simulink model "three_robot_cluster_all_primitives"  (R2024b)
settings: Solver=FixedStepDiscrete  StartTime=0.0  StopTime=60  FixedStep=0.1  MaxStep=0.1  RelTol=1e-3
libraries: neural x165, realtime_pacer_lib x1, simulink x1
(part 2 of 8)

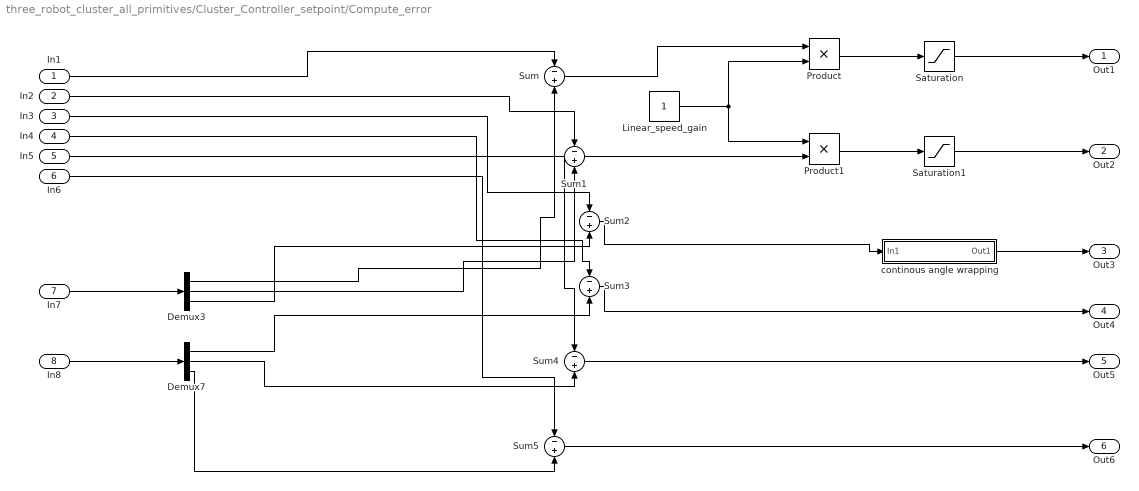
== system three_robot_cluster_all_primitives/Cluster_Controller_setpoint/Compute_error ==
  In1 : Inport
  In2 : Inport  Port=2
  In3 : Inport  Port=3
  In4 : Inport  Port=4
  In5 : Inport  Port=5
  In6 : Inport  Port=6
  In7 : Inport  Port=7
  In8 : Inport  Port=8
  Demux3 : Demux  Outputs=3
  Demux7 : Demux  Outputs=3
  Linear_speed_gain : Constant
  Product : Product
  Product1 : Product
  Saturation : Saturate  UpperLimit=0.3  LowerLimit=-0.3
  Saturation1 : Saturate  UpperLimit=0.3  LowerLimit=-0.3
  Sum{,1..5} (6 alike) : Sum  Inputs=-+
  continous angle wrapping : Subsystem
  Out1 : Outport
  Out2 : Outport  Port=2
  Out3 : Outport  Port=3
  Out4 : Outport  Port=4
  Out5 : Outport  Port=5
  Out6 : Outport  Port=6
  wires:
  In3/1 -> Sum2/1
  Demux3/2 -> Sum1/2
  Sum3/1 -> Out4/1
  In2/1 -> Sum1/1
  Demux3/3 -> Sum2/2
  Demux7/3 -> Sum5/2
  In8/1 -> Demux7/1
  Demux7/1 -> Sum3/2
  In1/1 -> Sum/1
  In5/1 -> Sum4/1
  Demux7/2 -> Sum4/2
  In6/1 -> Sum5/1
  Sum4/1 -> Out5/1
  Sum5/1 -> Out6/1
  Demux3/1 -> Sum/2
  In4/1 -> Sum3/1
  In7/1 -> Demux3/1
  Sum2/1 -> continous angle wrapping/1(In1)
  continous angle wrapping/1(Out1) -> Out3/1
  Sum/1 -> Product/1
  Linear_speed_gain/1 -> Product/2, Product1/1
  Sum1/1 -> Product1/2
  Saturation/1 -> Out1/1
  Product/1 -> Saturation/1
  Product1/1 -> Saturation1/1
  Saturation1/1 -> Out2/1

== system three_robot_cluster_all_primitives/Jacobian_primitive/Critical_point_predicter ==
  hue : Inport
  Sat : Inport  Port=2
  robot1 : Inport  Port=3
  robot2 : Inport  Port=4
  robot3 : Inport  Port=5
  Constant2 : Constant  Value=0
  Demux{,1..4} (5 alike) : Demux  Outputs=3
  Desired_set_point_Jacobian : ToWorkspace  VariableName=detected_critical_point  SampleTime=-1
  MATLAB Function : MATLAB Function  TreatAsAtomicUnit=on
  Sat_rescaling : Subsystem
  Subsystem : Subsystem
  Subsystem1 : Subsystem
  Subsystem2 : Subsystem
  Vector Concatenate : Concatenate
  x_desired : Outport
  y_desired : Outport  Port=2
  th_c_desired : Outport  Port=3
  wires:
  Vector Concatenate/1 -> Desired_set_point_Jacobian/1
  Constant2/1 -> th_c_desired/1
  Sat/1 -> Demux1/1
  hue/1 -> Demux/1
  Demux/1 -> Subsystem/1(hue)
  Demux/2 -> Subsystem1/1(hue)
  Demux/3 -> Subsystem2/1(hue)
  Demux1/1 -> Sat_rescaling/1(In1)
  Demux1/2 -> Sat_rescaling/2(In2)
  Demux1/3 -> Sat_rescaling/3(In3)
  Sat_rescaling/1(saturation) -> Subsystem/2(saturation)
  Sat_rescaling/2(saturation1) -> Subsystem1/2(saturation)
  Sat_rescaling/3(saturation2) -> Subsystem2/2(saturation)
  robot3/1 -> Demux4/1
  robot2/1 -> Demux3/1
  robot1/1 -> Demux2/1
  Subsystem/1(X_Component) -> MATLAB Function/3(u1)  "x_component"
  Subsystem/2(Y_Component) -> MATLAB Function/4(v1)  "y_component"
  Subsystem1/1(X_Component) -> MATLAB Function/7(u2)  "x_component"
  Subsystem1/2(Y_Component) -> MATLAB Function/8(v2)  "y_component"
  Subsystem2/1(X_Component) -> MATLAB Function/11(u3)  "x_component"
  Subsystem2/2(Y_Component) -> MATLAB Function/12(v3)  "y_component"
  Demux2/1 -> MATLAB Function/1(x1)
  Demux2/2 -> MATLAB Function/2(y1)
  Demux3/1 -> MATLAB Function/5(x2)
  Demux3/2 -> MATLAB Function/6(y2)
  Demux4/1 -> MATLAB Function/9(x3)
  Demux4/2 -> MATLAB Function/10(y3)
  MATLAB Function/1(x) -> Vector Concatenate/1, x_desired/1
  MATLAB Function/2(y) -> y_desired/1, Vector Concatenate/2

== system three_robot_cluster_all_primitives/Jacobian_primitive/formation_error ==
  a : Inport
  b : Inport  Port=2
  c : Inport  Port=3
  a,b,c desired : Inport  Port=4
  Demux7 : Demux  Outputs=3
  Sum3 : Sum  Inputs=-+
  Sum4 : Sum  Inputs=-+
  Sum5 : Sum  Inputs=-+
  a_err : Outport
  b_err : Outport  Port=2
  C_err : Outport  Port=3
  wires:
  Sum3/1 -> a_err/1
  Demux7/3 -> Sum5/2
  a,b,c desired/1 -> Demux7/1
  Demux7/1 -> Sum3/2
  b/1 -> Sum4/1
  Demux7/2 -> Sum4/2
  c/1 -> Sum5/1
  Sum4/1 -> b_err/1
  Sum5/1 -> C_err/1
  a/1 -> Sum3/1

== system three_robot_cluster_all_primitives/Jacobian_primitive/position_error ==
  x_c : Inport
  y_c : Inport  Port=2
  th_c : Inport  Port=3
  x,y,thC desired : Inport  Port=4
  Constant : Constant
  Demux7 : Demux  Outputs=3
  Product : Product
  Product1 : Product
  Saturation : Saturate  UpperLimit=0.3  LowerLimit=-0.3
  Saturation1 : Saturate  UpperLimit=0.3  LowerLimit=-0.3
  Sum3 : Sum  Inputs=-+
  Sum4 : Sum  Inputs=-+
  Sum5 : Sum  Inputs=-+
  thC_err : Outport
  xc_err : Outport  Port=2
  yc_err : Outport  Port=3
  wires:
  Demux7/3 -> Sum5/2
  x,y,thC desired/1 -> Demux7/1
  Demux7/1 -> Sum3/2
  y_c/1 -> Sum4/1
  Demux7/2 -> Sum4/2
  th_c/1 -> Sum5/1
  Sum5/1 -> thC_err/1
  x_c/1 -> Sum3/1
  Constant/1 -> Product1/1, Product/1
  Sum3/1 -> Product/2
  Sum4/1 -> Product1/2
  Saturation/1 -> xc_err/1
  Product/1 -> Saturation/1
  Saturation1/1 -> yc_err/1
  Product1/1 -> Saturation1/1

== system three_robot_cluster_all_primitives/RGB to HSV to vel - all robots/Hue Neural Network ==
  Input : Inport  PortDimensions=4
      mask Display: e = 0.06;c1 = [120 230 180]/255;c2 = ([120 230 180]+0)/(256+128);c3 = ([120 230 180]+128)/(256+128);patch([0 1 1 0],[0 0 1 1],c1);patch([0 1 1 1-e 1-e 0+e],[0 0 1 1-e 0+e 0+e],c2);patch([0 0 1 1-e 0+e 0+e],[0 1 1 1-e 1-e 0+e],c3);plot([0 1 1 0 0],[0 0 1 1 0]);
  Layer 1 : Subsystem
      mask Display: e = 0.06;c1 = [120 150 230]/255;c2 = ([120 150 230]+0)/383;c3 = ([120 150 230]+128)/383;patch([0 1 1 0],[0 0 1 1],c1);patch([0 1 1 1-e 1-e 0+e],[0 0 1 1-e 0+e 0+e],c2);patch([0 0 1 1-e 0+e 0+e],[0 1 1 1-e 1-e 0+e],c3);plot([0 1 1 0 0],[0 0 1 1 0]);
  Layer 2 : Subsystem
      mask Display: e = 0.06;c1 = [120 150 230]/255;c2 = ([120 150 230]+0)/383;c3 = ([120 150 230]+128)/383;patch([0 1 1 0],[0 0 1 1],c1);patch([0 1 1 1-e 1-e 0+e],[0 0 1 1-e 0+e 0+e],c2);patch([0 0 1 1-e 0+e 0+e],[0 1 1 1-e 1-e 0+e],c3);plot([0 1 1 0 0],[0 0 1 1 0]);
  Layer 3 : Subsystem
      mask Display: e = 0.06;c1 = [120 150 230]/255;c2 = ([120 150 230]+0)/383;c3 = ([120 150 230]+128)/383;patch([0 1 1 0],[0 0 1 1],c1);patch([0 1 1 1-e 1-e 0+e],[0 0 1 1-e 0+e 0+e],c2);patch([0 0 1 1-e 0+e 0+e],[0 1 1 1-e 1-e 0+e],c3);plot([0 1 1 0 0],[0 0 1 1 0]);
  Process Input 1 : Subsystem
      mask Display: e = 0.06;c1 = [120 150 230]/255;c2 = ([120 150 230]+0)/383;c3 = ([120 150 230]+128)/383;patch([0 1 1 0],[0 0 1 1],c1);patch([0 1 1 1-e 1-e 0+e],[0 0 1 1-e 0+e 0+e],c2);patch([0 0 1 1-e 0+e 0+e],[0 1 1 1-e 1-e 0+e],c3);plot([0 1 1 0 0],[0 0 1 1 0]);
  Process Output 1 : Subsystem
      mask Display: e = 0.06;c1 = [120 150 230]/255;c2 = ([120 150 230]+0)/383;c3 = ([120 150 230]+128)/383;patch([0 1 1 0],[0 0 1 1],c1);patch([0 1 1 1-e 1-e 0+e],[0 0 1 1-e 0+e 0+e],c2);patch([0 0 1 1-e 0+e 0+e],[0 1 1 1-e 1-e 0+e],c3);plot([0 1 1 0 0],[0 0 1 1 0]);
  Output : Outport  InitialOutput=[0;0]
      mask Display: e = 0.06;c1 = [120 230 180]/255;c2 = ([120 230 180]+0)/(256+128);c3 = ([120 230 180]+128)/(256+128);patch([0 1 1 0],[0 0 1 1],c1);patch([0 1 1 1-e 1-e 0+e],[0 0 1 1-e 0+e 0+e],c2);patch([0 0 1 1-e 0+e 0+e],[0 1 1 1-e 1-e 0+e],c3);plot([0 1 1 0 0],[0 0 1 1 0]);
  wires:
  Input/1 -> Process Input 1/1(x)
  Process Output 1/1(y) -> Output/1
  Process Input 1/1(p) -> Layer 1/1("p{1}")
  Layer 1/1("a{1}") -> [feedback1]
  [feedback1] -> Layer 2/1("a{1} ")
  Layer 2/1("a{2}") -> [feedback2]
  [feedback2] -> Layer 3/1("a{2} ")
  Layer 3/1("a{3}") -> Process Output 1/1(a)

== system three_robot_cluster_all_primitives/RGB to HSV to vel - all robots/Sat Neural Network ==
  Input : Inport  PortDimensions=4
      mask Display: e = 0.06;c1 = [120 230 180]/255;c2 = ([120 230 180]+0)/(256+128);c3 = ([120 230 180]+128)/(256+128);patch([0 1 1 0],[0 0 1 1],c1);patch([0 1 1 1-e 1-e 0+e],[0 0 1 1-e 0+e 0+e],c2);patch([0 0 1 1-e 0+e 0+e],[0 1 1 1-e 1-e 0+e],c3);plot([0 1 1 0 0],[0 0 1 1 0]);
  Layer 1 : Subsystem
      mask Display: e = 0.06;c1 = [120 150 230]/255;c2 = ([120 150 230]+0)/383;c3 = ([120 150 230]+128)/383;patch([0 1 1 0],[0 0 1 1],c1);patch([0 1 1 1-e 1-e 0+e],[0 0 1 1-e 0+e 0+e],c2);patch([0 0 1 1-e 0+e 0+e],[0 1 1 1-e 1-e 0+e],c3);plot([0 1 1 0 0],[0 0 1 1 0]);
  Layer 2 : Subsystem
      mask Display: e = 0.06;c1 = [120 150 230]/255;c2 = ([120 150 230]+0)/383;c3 = ([120 150 230]+128)/383;patch([0 1 1 0],[0 0 1 1],c1);patch([0 1 1 1-e 1-e 0+e],[0 0 1 1-e 0+e 0+e],c2);patch([0 0 1 1-e 0+e 0+e],[0 1 1 1-e 1-e 0+e],c3);plot([0 1 1 0 0],[0 0 1 1 0]);
  Layer 3 : Subsystem
      mask Display: e = 0.06;c1 = [120 150 230]/255;c2 = ([120 150 230]+0)/383;c3 = ([120 150 230]+128)/383;patch([0 1 1 0],[0 0 1 1],c1);patch([0 1 1 1-e 1-e 0+e],[0 0 1 1-e 0+e 0+e],c2);patch([0 0 1 1-e 0+e 0+e],[0 1 1 1-e 1-e 0+e],c3);plot([0 1 1 0 0],[0 0 1 1 0]);
  Process Input 1 : Subsystem
      mask Display: e = 0.06;c1 = [120 150 230]/255;c2 = ([120 150 230]+0)/383;c3 = ([120 150 230]+128)/383;patch([0 1 1 0],[0 0 1 1],c1);patch([0 1 1 1-e 1-e 0+e],[0 0 1 1-e 0+e 0+e],c2);patch([0 0 1 1-e 0+e 0+e],[0 1 1 1-e 1-e 0+e],c3);plot([0 1 1 0 0],[0 0 1 1 0]);
  Process Output 1 : Subsystem
      mask Display: e = 0.06;c1 = [120 150 230]/255;c2 = ([120 150 230]+0)/383;c3 = ([120 150 230]+128)/383;patch([0 1 1 0],[0 0 1 1],c1);patch([0 1 1 1-e 1-e 0+e],[0 0 1 1-e 0+e 0+e],c2);patch([0 0 1 1-e 0+e 0+e],[0 1 1 1-e 1-e 0+e],c3);plot([0 1 1 0 0],[0 0 1 1 0]);
  Output : Outport  InitialOutput=0
      mask Display: e = 0.06;c1 = [120 230 180]/255;c2 = ([120 230 180]+0)/(256+128);c3 = ([120 230 180]+128)/(256+128);patch([0 1 1 0],[0 0 1 1],c1);patch([0 1 1 1-e 1-e 0+e],[0 0 1 1-e 0+e 0+e],c2);patch([0 0 1 1-e 0+e 0+e],[0 1 1 1-e 1-e 0+e],c3);plot([0 1 1 0 0],[0 0 1 1 0]);
  wires:
  Input/1 -> Process Input 1/1(x)
  Process Output 1/1(y) -> Output/1
  Process Input 1/1(p) -> Layer 1/1("p{1}")
  Layer 1/1("a{1}") -> [feedback1]
  [feedback1] -> Layer 2/1("a{1} ")
  Layer 2/1("a{2}") -> [feedback2]
  [feedback2] -> Layer 3/1("a{2} ")
  Layer 3/1("a{3}") -> Process Output 1/1(a)

== system three_robot_cluster_all_primitives/RGB to HSV to vel - all robots1/Hue Neural Network ==
  Input : Inport  PortDimensions=4
      mask Display: e = 0.06;c1 = [120 230 180]/255;c2 = ([120 230 180]+0)/(256+128);c3 = ([120 230 180]+128)/(256+128);patch([0 1 1 0],[0 0 1 1],c1);patch([0 1 1 1-e 1-e 0+e],[0 0 1 1-e 0+e 0+e],c2);patch([0 0 1 1-e 0+e 0+e],[0 1 1 1-e 1-e 0+e],c3);plot([0 1 1 0 0],[0 0 1 1 0]);
  Layer 1 : Subsystem
      mask Display: e = 0.06;c1 = [120 150 230]/255;c2 = ([120 150 230]+0)/383;c3 = ([120 150 230]+128)/383;patch([0 1 1 0],[0 0 1 1],c1);patch([0 1 1 1-e 1-e 0+e],[0 0 1 1-e 0+e 0+e],c2);patch([0 0 1 1-e 0+e 0+e],[0 1 1 1-e 1-e 0+e],c3);plot([0 1 1 0 0],[0 0 1 1 0]);
  Layer 2 : Subsystem
      mask Display: e = 0.06;c1 = [120 150 230]/255;c2 = ([120 150 230]+0)/383;c3 = ([120 150 230]+128)/383;patch([0 1 1 0],[0 0 1 1],c1);patch([0 1 1 1-e 1-e 0+e],[0 0 1 1-e 0+e 0+e],c2);patch([0 0 1 1-e 0+e 0+e],[0 1 1 1-e 1-e 0+e],c3);plot([0 1 1 0 0],[0 0 1 1 0]);
  Layer 3 : Subsystem
      mask Display: e = 0.06;c1 = [120 150 230]/255;c2 = ([120 150 230]+0)/383;c3 = ([120 150 230]+128)/383;patch([0 1 1 0],[0 0 1 1],c1);patch([0 1 1 1-e 1-e 0+e],[0 0 1 1-e 0+e 0+e],c2);patch([0 0 1 1-e 0+e 0+e],[0 1 1 1-e 1-e 0+e],c3);plot([0 1 1 0 0],[0 0 1 1 0]);
  Process Input 1 : Subsystem
      mask Display: e = 0.06;c1 = [120 150 230]/255;c2 = ([120 150 230]+0)/383;c3 = ([120 150 230]+128)/383;patch([0 1 1 0],[0 0 1 1],c1);patch([0 1 1 1-e 1-e 0+e],[0 0 1 1-e 0+e 0+e],c2);patch([0 0 1 1-e 0+e 0+e],[0 1 1 1-e 1-e 0+e],c3);plot([0 1 1 0 0],[0 0 1 1 0]);
  Process Output 1 : Subsystem
      mask Display: e = 0.06;c1 = [120 150 230]/255;c2 = ([120 150 230]+0)/383;c3 = ([120 150 230]+128)/383;patch([0 1 1 0],[0 0 1 1],c1);patch([0 1 1 1-e 1-e 0+e],[0 0 1 1-e 0+e 0+e],c2);patch([0 0 1 1-e 0+e 0+e],[0 1 1 1-e 1-e 0+e],c3);plot([0 1 1 0 0],[0 0 1 1 0]);
  Output : Outport  InitialOutput=[0;0]
      mask Display: e = 0.06;c1 = [120 230 180]/255;c2 = ([120 230 180]+0)/(256+128);c3 = ([120 230 180]+128)/(256+128);patch([0 1 1 0],[0 0 1 1],c1);patch([0 1 1 1-e 1-e 0+e],[0 0 1 1-e 0+e 0+e],c2);patch([0 0 1 1-e 0+e 0+e],[0 1 1 1-e 1-e 0+e],c3);plot([0 1 1 0 0],[0 0 1 1 0]);
  wires:
  Input/1 -> Process Input 1/1(x)
  Process Output 1/1(y) -> Output/1
  Process Input 1/1(p) -> Layer 1/1("p{1}")
  Layer 1/1("a{1}") -> [feedback1]
  [feedback1] -> Layer 2/1("a{1} ")
  Layer 2/1("a{2}") -> [feedback2]
  [feedback2] -> Layer 3/1("a{2} ")
  Layer 3/1("a{3}") -> Process Output 1/1(a)

== system three_robot_cluster_all_primitives/RGB to HSV to vel - all robots1/Sat Neural Network ==
  Input : Inport  PortDimensions=4
      mask Display: e = 0.06;c1 = [120 230 180]/255;c2 = ([120 230 180]+0)/(256+128);c3 = ([120 230 180]+128)/(256+128);patch([0 1 1 0],[0 0 1 1],c1);patch([0 1 1 1-e 1-e 0+e],[0 0 1 1-e 0+e 0+e],c2);patch([0 0 1 1-e 0+e 0+e],[0 1 1 1-e 1-e 0+e],c3);plot([0 1 1 0 0],[0 0 1 1 0]);
  Layer 1 : Subsystem
      mask Display: e = 0.06;c1 = [120 150 230]/255;c2 = ([120 150 230]+0)/383;c3 = ([120 150 230]+128)/383;patch([0 1 1 0],[0 0 1 1],c1);patch([0 1 1 1-e 1-e 0+e],[0 0 1 1-e 0+e 0+e],c2);patch([0 0 1 1-e 0+e 0+e],[0 1 1 1-e 1-e 0+e],c3);plot([0 1 1 0 0],[0 0 1 1 0]);
  Layer 2 : Subsystem
      mask Display: e = 0.06;c1 = [120 150 230]/255;c2 = ([120 150 230]+0)/383;c3 = ([120 150 230]+128)/383;patch([0 1 1 0],[0 0 1 1],c1);patch([0 1 1 1-e 1-e 0+e],[0 0 1 1-e 0+e 0+e],c2);patch([0 0 1 1-e 0+e 0+e],[0 1 1 1-e 1-e 0+e],c3);plot([0 1 1 0 0],[0 0 1 1 0]);
  Layer 3 : Subsystem
      mask Display: e = 0.06;c1 = [120 150 230]/255;c2 = ([120 150 230]+0)/383;c3 = ([120 150 230]+128)/383;patch([0 1 1 0],[0 0 1 1],c1);patch([0 1 1 1-e 1-e 0+e],[0 0 1 1-e 0+e 0+e],c2);patch([0 0 1 1-e 0+e 0+e],[0 1 1 1-e 1-e 0+e],c3);plot([0 1 1 0 0],[0 0 1 1 0]);
  Process Input 1 : Subsystem
      mask Display: e = 0.06;c1 = [120 150 230]/255;c2 = ([120 150 230]+0)/383;c3 = ([120 150 230]+128)/383;patch([0 1 1 0],[0 0 1 1],c1);patch([0 1 1 1-e 1-e 0+e],[0 0 1 1-e 0+e 0+e],c2);patch([0 0 1 1-e 0+e 0+e],[0 1 1 1-e 1-e 0+e],c3);plot([0 1 1 0 0],[0 0 1 1 0]);
  Process Output 1 : Subsystem
      mask Display: e = 0.06;c1 = [120 150 230]/255;c2 = ([120 150 230]+0)/383;c3 = ([120 150 230]+128)/383;patch([0 1 1 0],[0 0 1 1],c1);patch([0 1 1 1-e 1-e 0+e],[0 0 1 1-e 0+e 0+e],c2);patch([0 0 1 1-e 0+e 0+e],[0 1 1 1-e 1-e 0+e],c3);plot([0 1 1 0 0],[0 0 1 1 0]);
  Output : Outport  InitialOutput=0
      mask Display: e = 0.06;c1 = [120 230 180]/255;c2 = ([120 230 180]+0)/(256+128);c3 = ([120 230 180]+128)/(256+128);patch([0 1 1 0],[0 0 1 1],c1);patch([0 1 1 1-e 1-e 0+e],[0 0 1 1-e 0+e 0+e],c2);patch([0 0 1 1-e 0+e 0+e],[0 1 1 1-e 1-e 0+e],c3);plot([0 1 1 0 0],[0 0 1 1 0]);
  wires:
  Input/1 -> Process Input 1/1(x)
  Process Output 1/1(y) -> Output/1
  Process Input 1/1(p) -> Layer 1/1("p{1}")
  Layer 1/1("a{1}") -> [feedback1]
  [feedback1] -> Layer 2/1("a{1} ")
  Layer 2/1("a{2}") -> [feedback2]
  [feedback2] -> Layer 3/1("a{2} ")
  Layer 3/1("a{3}") -> Process Output 1/1(a)

== system three_robot_cluster_all_primitives/RGB to HSV to vel - all robots2/Hue Neural Network ==
  Input : Inport  PortDimensions=4
      mask Display: e = 0.06;c1 = [120 230 180]/255;c2 = ([120 230 180]+0)/(256+128);c3 = ([120 230 180]+128)/(256+128);patch([0 1 1 0],[0 0 1 1],c1);patch([0 1 1 1-e 1-e 0+e],[0 0 1 1-e 0+e 0+e],c2);patch([0 0 1 1-e 0+e 0+e],[0 1 1 1-e 1-e 0+e],c3);plot([0 1 1 0 0],[0 0 1 1 0]);
  Layer 1 : Subsystem
      mask Display: e = 0.06;c1 = [120 150 230]/255;c2 = ([120 150 230]+0)/383;c3 = ([120 150 230]+128)/383;patch([0 1 1 0],[0 0 1 1],c1);patch([0 1 1 1-e 1-e 0+e],[0 0 1 1-e 0+e 0+e],c2);patch([0 0 1 1-e 0+e 0+e],[0 1 1 1-e 1-e 0+e],c3);plot([0 1 1 0 0],[0 0 1 1 0]);
  Layer 2 : Subsystem
      mask Display: e = 0.06;c1 = [120 150 230]/255;c2 = ([120 150 230]+0)/383;c3 = ([120 150 230]+128)/383;patch([0 1 1 0],[0 0 1 1],c1);patch([0 1 1 1-e 1-e 0+e],[0 0 1 1-e 0+e 0+e],c2);patch([0 0 1 1-e 0+e 0+e],[0 1 1 1-e 1-e 0+e],c3);plot([0 1 1 0 0],[0 0 1 1 0]);
  Layer 3 : Subsystem
      mask Display: e = 0.06;c1 = [120 150 230]/255;c2 = ([120 150 230]+0)/383;c3 = ([120 150 230]+128)/383;patch([0 1 1 0],[0 0 1 1],c1);patch([0 1 1 1-e 1-e 0+e],[0 0 1 1-e 0+e 0+e],c2);patch([0 0 1 1-e 0+e 0+e],[0 1 1 1-e 1-e 0+e],c3);plot([0 1 1 0 0],[0 0 1 1 0]);
  Process Input 1 : Subsystem
      mask Display: e = 0.06;c1 = [120 150 230]/255;c2 = ([120 150 230]+0)/383;c3 = ([120 150 230]+128)/383;patch([0 1 1 0],[0 0 1 1],c1);patch([0 1 1 1-e 1-e 0+e],[0 0 1 1-e 0+e 0+e],c2);patch([0 0 1 1-e 0+e 0+e],[0 1 1 1-e 1-e 0+e],c3);plot([0 1 1 0 0],[0 0 1 1 0]);
  Process Output 1 : Subsystem
      mask Display: e = 0.06;c1 = [120 150 230]/255;c2 = ([120 150 230]+0)/383;c3 = ([120 150 230]+128)/383;patch([0 1 1 0],[0 0 1 1],c1);patch([0 1 1 1-e 1-e 0+e],[0 0 1 1-e 0+e 0+e],c2);patch([0 0 1 1-e 0+e 0+e],[0 1 1 1-e 1-e 0+e],c3);plot([0 1 1 0 0],[0 0 1 1 0]);
  Output : Outport  InitialOutput=[0;0]
      mask Display: e = 0.06;c1 = [120 230 180]/255;c2 = ([120 230 180]+0)/(256+128);c3 = ([120 230 180]+128)/(256+128);patch([0 1 1 0],[0 0 1 1],c1);patch([0 1 1 1-e 1-e 0+e],[0 0 1 1-e 0+e 0+e],c2);patch([0 0 1 1-e 0+e 0+e],[0 1 1 1-e 1-e 0+e],c3);plot([0 1 1 0 0],[0 0 1 1 0]);
  wires:
  Input/1 -> Process Input 1/1(x)
  Process Output 1/1(y) -> Output/1
  Process Input 1/1(p) -> Layer 1/1("p{1}")
  Layer 1/1("a{1}") -> [feedback1]
  [feedback1] -> Layer 2/1("a{1} ")
  Layer 2/1("a{2}") -> [feedback2]
  [feedback2] -> Layer 3/1("a{2} ")
  Layer 3/1("a{3}") -> Process Output 1/1(a)

== system three_robot_cluster_all_primitives/RGB to HSV to vel - all robots2/Sat Neural Network ==
  Input : Inport  PortDimensions=4
      mask Display: e = 0.06;c1 = [120 230 180]/255;c2 = ([120 230 180]+0)/(256+128);c3 = ([120 230 180]+128)/(256+128);patch([0 1 1 0],[0 0 1 1],c1);patch([0 1 1 1-e 1-e 0+e],[0 0 1 1-e 0+e 0+e],c2);patch([0 0 1 1-e 0+e 0+e],[0 1 1 1-e 1-e 0+e],c3);plot([0 1 1 0 0],[0 0 1 1 0]);
  Layer 1 : Subsystem
      mask Display: e = 0.06;c1 = [120 150 230]/255;c2 = ([120 150 230]+0)/383;c3 = ([120 150 230]+128)/383;patch([0 1 1 0],[0 0 1 1],c1);patch([0 1 1 1-e 1-e 0+e],[0 0 1 1-e 0+e 0+e],c2);patch([0 0 1 1-e 0+e 0+e],[0 1 1 1-e 1-e 0+e],c3);plot([0 1 1 0 0],[0 0 1 1 0]);
  Layer 2 : Subsystem
      mask Display: e = 0.06;c1 = [120 150 230]/255;c2 = ([120 150 230]+0)/383;c3 = ([120 150 230]+128)/383;patch([0 1 1 0],[0 0 1 1],c1);patch([0 1 1 1-e 1-e 0+e],[0 0 1 1-e 0+e 0+e],c2);patch([0 0 1 1-e 0+e 0+e],[0 1 1 1-e 1-e 0+e],c3);plot([0 1 1 0 0],[0 0 1 1 0]);
  Layer 3 : Subsystem
      mask Display: e = 0.06;c1 = [120 150 230]/255;c2 = ([120 150 230]+0)/383;c3 = ([120 150 230]+128)/383;patch([0 1 1 0],[0 0 1 1],c1);patch([0 1 1 1-e 1-e 0+e],[0 0 1 1-e 0+e 0+e],c2);patch([0 0 1 1-e 0+e 0+e],[0 1 1 1-e 1-e 0+e],c3);plot([0 1 1 0 0],[0 0 1 1 0]);
  Process Input 1 : Subsystem
      mask Display: e = 0.06;c1 = [120 150 230]/255;c2 = ([120 150 230]+0)/383;c3 = ([120 150 230]+128)/383;patch([0 1 1 0],[0 0 1 1],c1);patch([0 1 1 1-e 1-e 0+e],[0 0 1 1-e 0+e 0+e],c2);patch([0 0 1 1-e 0+e 0+e],[0 1 1 1-e 1-e 0+e],c3);plot([0 1 1 0 0],[0 0 1 1 0]);
  Process Output 1 : Subsystem
      mask Display: e = 0.06;c1 = [120 150 230]/255;c2 = ([120 150 230]+0)/383;c3 = ([120 150 230]+128)/383;patch([0 1 1 0],[0 0 1 1],c1);patch([0 1 1 1-e 1-e 0+e],[0 0 1 1-e 0+e 0+e],c2);patch([0 0 1 1-e 0+e 0+e],[0 1 1 1-e 1-e 0+e],c3);plot([0 1 1 0 0],[0 0 1 1 0]);
  Output : Outport  InitialOutput=0
      mask Display: e = 0.06;c1 = [120 230 180]/255;c2 = ([120 230 180]+0)/(256+128);c3 = ([120 230 180]+128)/(256+128);patch([0 1 1 0],[0 0 1 1],c1);patch([0 1 1 1-e 1-e 0+e],[0 0 1 1-e 0+e 0+e],c2);patch([0 0 1 1-e 0+e 0+e],[0 1 1 1-e 1-e 0+e],c3);plot([0 1 1 0 0],[0 0 1 1 0]);
  wires:
  Input/1 -> Process Input 1/1(x)
  Process Output 1/1(y) -> Output/1
  Process Input 1/1(p) -> Layer 1/1("p{1}")
  Layer 1/1("a{1}") -> [feedback1]
  [feedback1] -> Layer 2/1("a{1} ")
  Layer 2/1("a{2}") -> [feedback2]
  [feedback2] -> Layer 3/1("a{2} ")
  Layer 3/1("a{3}") -> Process Output 1/1(a)

== system three_robot_cluster_all_primitives/vector2scalar_mag_steepest_ascent/3_robot HSV to vector ==
  Sat : Inport
  Robot_1_pose : Inport  Port=2
  robot_2_pose : Inport  Port=3
  robot_3_pose : Inport  Port=4
  Constant2 : Constant  Value=0
  Demux{,1..3} (4 alike) : Demux  Outputs=3
  Desired_velocities_new_primitve : ToWorkspace  VariableName=desired_velocities_gradient_descent  SampleTime=-1
  MATLAB Function : MATLAB Function  TreatAsAtomicUnit=on
  Scope : Scope  NumInputPorts=2
  Scope1 : Scope  NumInputPorts=2
  Scope2 : Scope  NumInputPorts=3
  Vector Concatenate : Concatenate  NumInputs=3
  y_velocity : Outport
  x_velocity : Outport  Port=2
  th_c velocity : Outport  Port=3
  wires:
  Vector Concatenate/1 -> Desired_velocities_new_primitve/1
  Constant2/1 -> th_c velocity/1, Vector Concatenate/3
  Sat/1 -> Demux/1
  Robot_1_pose/1 -> Demux1/1
  robot_2_pose/1 -> Demux2/1
  robot_3_pose/1 -> Demux3/1
  Demux1/1 -> Scope1/1, MATLAB Function/1(x1)
  Demux1/2 -> MATLAB Function/2(y1), Scope1/2
  Demux/1 -> Scope2/1, MATLAB Function/3(z1)
  Demux2/1 -> MATLAB Function/4(x2)
  Demux2/2 -> MATLAB Function/5(y2)
  Demux/2 -> Scope2/2, MATLAB Function/6(z2)
  Demux3/1 -> MATLAB Function/7(x3)
  Demux3/2 -> MATLAB Function/8(y3)
  Demux/3 -> Scope2/3, MATLAB Function/9(z3)
  MATLAB Function/1(x) -> Scope/1, x_velocity/1, Vector Concatenate/1
  MATLAB Function/2(y) -> Scope/2, y_velocity/1, Vector Concatenate/2

== system three_robot_cluster_all_primitives/vector2scalar_mag_steepest_ascent/formation_error ==
  a : Inport
  b : Inport  Port=2
  c : Inport  Port=3
  a,b,c desired : Inport  Port=4
  Demux7 : Demux  Outputs=3
  Sum3 : Sum  Inputs=-+
  Sum4 : Sum  Inputs=-+
  Sum5 : Sum  Inputs=-+
  Out4 : Outport
  Out5 : Outport  Port=2
  Out6 : Outport  Port=3
  wires:
  Sum3/1 -> Out4/1
  Demux7/3 -> Sum5/2
  a,b,c desired/1 -> Demux7/1
  Demux7/1 -> Sum3/2
  b/1 -> Sum4/1
  Demux7/2 -> Sum4/2
  c/1 -> Sum5/1
  Sum4/1 -> Out5/1
  Sum5/1 -> Out6/1
  a/1 -> Sum3/1

== system three_robot_cluster_all_primitives/vector2scalar_mag_steepest_descent/3_robot HSV to vector ==
  Sat : Inport
  Robot_1_pose : Inport  Port=2
  robot_2_pose : Inport  Port=3
  robot_3_pose : Inport  Port=4
  Constant2 : Constant  Value=0
  Demux{,1..3} (4 alike) : Demux  Outputs=3
  MATLAB Function : MATLAB Function  TreatAsAtomicUnit=on
  Scope : Scope  NumInputPorts=2
  Scope1 : Scope  NumInputPorts=2
  Scope2 : Scope  NumInputPorts=2
  x_velocity : Outport
  th_c velocity : Outport  Port=2
  y_velocity : Outport  Port=3
  wires:
  Constant2/1 -> th_c velocity/1
  Sat/1 -> Demux/1
  Robot_1_pose/1 -> Demux1/1
  robot_2_pose/1 -> Demux2/1
  robot_3_pose/1 -> Demux3/1
  Demux1/1 -> Scope1/1, MATLAB Function/1(x1)
  Demux1/2 -> MATLAB Function/2(y1), Scope1/2
  Demux/1 -> Scope2/1, MATLAB Function/3(z1)
  Demux2/1 -> MATLAB Function/4(x2)
  Demux2/2 -> MATLAB Function/5(y2)
  Demux/2 -> Scope2/2, MATLAB Function/6(z2)
  Demux3/1 -> MATLAB Function/7(x3)
  Demux3/2 -> MATLAB Function/8(y3)
  Demux/3 -> MATLAB Function/9(z3)
  MATLAB Function/1(x) -> Scope/1, x_velocity/1
  MATLAB Function/2(y) -> y_velocity/1, Scope/2

== system three_robot_cluster_all_primitives/vector2scalar_mag_steepest_descent/formation_error ==
  a : Inport
  b : Inport  Port=2
  c : Inport  Port=3
  a,b,c desired : Inport  Port=4
  Demux7 : Demux  Outputs=3
  Sum3 : Sum  Inputs=-+
  Sum4 : Sum  Inputs=-+
  Sum5 : Sum  Inputs=-+
  Out4 : Outport
  Out5 : Outport  Port=2
  Out6 : Outport  Port=3
  wires:
  Sum3/1 -> Out4/1
  Demux7/3 -> Sum5/2
  a,b,c desired/1 -> Demux7/1
  Demux7/1 -> Sum3/2
  b/1 -> Sum4/1
  Demux7/2 -> Sum4/2
  c/1 -> Sum5/1
  Sum4/1 -> Out5/1
  Sum5/1 -> Out6/1
  a/1 -> Sum3/1

== system three_robot_cluster_all_primitives/vector_sum/3_robot HSV to vector ==
  hue : Inport
  Sat : Inport  Port=2
  Constant2 : Constant  Value=0
  Demux : Demux  Outputs=3
  Demux1 : Demux  Outputs=3
  Desired_velocities_dir__and_mag_follower : ToWorkspace  VariableName=desired_velocities  SampleTime=-1
  Product3 : Product
  Product4 : Product
  Product5 : Product
  Sat_rescaling : Subsystem
  Subsystem : Subsystem
  Subsystem1 : Subsystem
  Subsystem2 : Subsystem
  Sum : Sum  Inputs=|+++
  Sum1 : Sum  Inputs=|+++
  Vector Concatenate : Concatenate  NumInputs=3
  X : Display
  Y : Display
  sat_to_velocity_scaler : Constant
  z-Direction Reverser : Constant
  y_velocity : Outport
  x_velocity : Outport  Port=2
  th_c velocity : Outport  Port=3
  wires:
  Sum/1 -> Product5/1
  Sum1/1 -> Product3/1
  Vector Concatenate/1 -> Desired_velocities_dir__and_mag_follower/1
  z-Direction Reverser/1 -> Product3/2
  Product3/1 -> Product4/1
  Product5/1 -> Vector Concatenate/1, x_velocity/1, X/1
  Constant2/1 -> Vector Concatenate/3, th_c velocity/1
  Product4/1 -> y_velocity/1, Y/1, Vector Concatenate/2
  sat_to_velocity_scaler/1 -> Product5/2, Product4/2
  Sat/1 -> Demux1/1
  hue/1 -> Demux/1
  Demux/1 -> Subsystem/1(hue)
  Subsystem/1(X_Component) -> Sum/1  "x_component"
  Subsystem/2(Y_Component) -> Sum1/1  "y_component"
  Demux/2 -> Subsystem1/1(hue)
  Demux/3 -> Subsystem2/1(hue)
  Subsystem1/1(X_Component) -> Sum/2  "x_component"
  Subsystem1/2(Y_Component) -> Sum1/2  "y_component"
  Subsystem2/1(X_Component) -> Sum/3  "x_component"
  Subsystem2/2(Y_Component) -> Sum1/3  "y_component"
  Demux1/1 -> Sat_rescaling/1(In1)
  Demux1/2 -> Sat_rescaling/2(In2)
  Demux1/3 -> Sat_rescaling/3(In3)
  Sat_rescaling/1(saturation) -> Subsystem/2(saturation)
  Sat_rescaling/2(saturation1) -> Subsystem1/2(saturation)
  Sat_rescaling/3(saturation2) -> Subsystem2/2(saturation)

== system three_robot_cluster_all_primitives/vector_sum/formation_error ==
  a : Inport
  b : Inport  Port=2
  c : Inport  Port=3
  a,b,c desired : Inport  Port=4
  Demux7 : Demux  Outputs=3
  Sum3 : Sum  Inputs=-+
  Sum4 : Sum  Inputs=-+
  Sum5 : Sum  Inputs=-+
  Out4 : Outport
  Out5 : Outport  Port=2
  Out6 : Outport  Port=3
  wires:
  Sum3/1 -> Out4/1
  Demux7/3 -> Sum5/2
  a,b,c desired/1 -> Demux7/1
  Demux7/1 -> Sum3/2
  b/1 -> Sum4/1
  Demux7/2 -> Sum4/2
  c/1 -> Sum5/1
  Sum4/1 -> Out5/1
  Sum5/1 -> Out6/1
  a/1 -> Sum3/1

== system three_robot_cluster_all_primitives/Cluster_Controller_setpoint/Compute_error/continous angle wrapping ==
  In1 : Inport
  Constant : Constant  Value=pi
  Constant1 : Constant  Value=2*pi
  Math Function : Math  Operator=mod  SignedPower=on
  Sum6 : Sum
  Sum7 : Sum  Inputs=-+
  Out1 : Outport
  wires:
  In1/1 -> Sum6/2
  Math Function/1 -> Sum7/2
  Constant/1 -> Sum7/1, Sum6/1
  Sum6/1 -> Math Function/1
  Constant1/1 -> Math Function/2
  Sum7/1 -> Out1/1

== system three_robot_cluster_all_primitives/Jacobian_primitive/Critical_point_predicter/Sat_rescaling ==
  In1 : Inport
  In2 : Inport  Port=2
  In3 : Inport  Port=3
  Saturation_clipped_and_rescaled : Subsystem
  Saturation_clipped_and_rescaled1 : Subsystem
  Saturation_clipped_and_rescaled2 : Subsystem
  saturation : Outport
  saturation1 : Outport  Port=2
  saturation2 : Outport  Port=3
  wires:
  Saturation_clipped_and_rescaled2/1(saturation) -> saturation2/1
  Saturation_clipped_and_rescaled1/1(saturation) -> saturation1/1
  In1/1 -> Saturation_clipped_and_rescaled/1(In1)
  In2/1 -> Saturation_clipped_and_rescaled1/1(In1)
  In3/1 -> Saturation_clipped_and_rescaled2/1(In1)
  Saturation_clipped_and_rescaled/1(saturation) -> saturation/1

== system three_robot_cluster_all_primitives/Jacobian_primitive/Critical_point_predicter/Subsystem ==
  hue : Inport
  saturation : Inport  Port=2
  Product : Product
  Product1 : Product
  Product2 : Product
  Trigonometric Function : Trigonometry
  Trigonometric Function1 : Trigonometry  Operator=cos
  opencv_2_360_converter : Constant  Value=2*pi
  X_Component : Outport
  Y_Component : Outport  Port=2
  wires:
  Product2/1 -> Y_Component/1
  Trigonometric Function1/1 -> Product2/1
  Product/1 -> Trigonometric Function1/1, Trigonometric Function/1
  Product1/1 -> X_Component/1
  hue/1 -> Product/1
  opencv_2_360_converter/1 -> Product/2
  Trigonometric Function/1 -> Product1/1
  saturation/1 -> Product2/2, Product1/2

== system three_robot_cluster_all_primitives/Jacobian_primitive/Critical_point_predicter/Subsystem1 ==
  hue : Inport
  saturation : Inport  Port=2
  Product : Product
  Product1 : Product
  Product2 : Product
  Trigonometric Function : Trigonometry
  Trigonometric Function1 : Trigonometry  Operator=cos
  opencv_2_360_converter : Constant  Value=2*pi
  X_Component : Outport
  Y_Component : Outport  Port=2
  wires:
  Product2/1 -> Y_Component/1
  Trigonometric Function1/1 -> Product2/1
  Product/1 -> Trigonometric Function1/1, Trigonometric Function/1
  Product1/1 -> X_Component/1
  hue/1 -> Product/1
  opencv_2_360_converter/1 -> Product/2
  Trigonometric Function/1 -> Product1/1
  saturation/1 -> Product2/2, Product1/2

== system three_robot_cluster_all_primitives/Jacobian_primitive/Critical_point_predicter/Subsystem2 ==
  hue : Inport
  saturation : Inport  Port=2
  Product : Product
  Product1 : Product
  Product2 : Product
  Trigonometric Function : Trigonometry
  Trigonometric Function1 : Trigonometry  Operator=cos
  opencv_2_360_converter : Constant  Value=2*pi
  X_Component : Outport
  Y_Component : Outport  Port=2
  wires:
  Product2/1 -> Y_Component/1
  Trigonometric Function1/1 -> Product2/1
  Product/1 -> Trigonometric Function1/1, Trigonometric Function/1
  Product1/1 -> X_Component/1
  hue/1 -> Product/1
  opencv_2_360_converter/1 -> Product/2
  Trigonometric Function/1 -> Product1/1
  saturation/1 -> Product2/2, Product1/2

== system three_robot_cluster_all_primitives/RGB to HSV to vel - all robots/Hue Neural Network/Layer 1 ==
  "p{1}" : Inport  PortDimensions=4
      mask Display: e = 0.06;c1 = [120 230 180]/255;c2 = ([120 230 180]+0)/(256+128);c3 = ([120 230 180]+128)/(256+128);patch([0 1 1 0],[0 0 1 1],c1);patch([0 1 1 1-e 1-e 0+e],[0 0 1 1-e 0+e 0+e],c2);patch([0 0 1 1-e 0+e 0+e],[0 1 1 1-e 1-e 0+e],c3);plot([0 1 1 0 0],[0 0 1 1 0]);
  Delays 1 : Subsystem
      mask Display: e = 0.06;c1 = [120 150 230]/255;c2 = ([120 150 230]+0)/383;c3 = ([120 150 230]+128)/383;patch([0 1 1 0],[0 0 1 1],c1);patch([0 1 1 1-e 1-e 0+e],[0 0 1 1-e 0+e 0+e],c2);patch([0 0 1 1-e 0+e 0+e],[0 1 1 1-e 1-e 0+e],c3);plot([0 1 1 0 0],[0 0 1 1 0]);disp('0');
  "IW{1,1}" : Subsystem
      mask Display: e = 0.06;c1 = [120 150 230]/255;c2 = ([120 150 230]+0)/383;c3 = ([120 150 230]+128)/383;patch([0 1 1 0],[0 0 1 1],c1);patch([0 1 1 1-e 1-e 0+e],[0 0 1 1-e 0+e 0+e],c2);patch([0 0 1 1-e 0+e 0+e],[0 1 1 1-e 1-e 0+e],c3);plot([0 1 1 0 0],[0 0 1 1 0]);disp('W');
  "b{1}" : Constant  Value=[-0.2383253726449501008755049724641139619052410125732421875;6.85787862695611494245895300991833209991455078125;0.0373737753295186048152487501283758319914340972900390625;0.998298703222104233390155059169046580791473388671875;2.681072744199842095014219012227840721607208251953125;7.021952292197259026806932524777948856353759765625;-0.389355131072435967087841390821267850697040557861328125;-55.97545927395623266420443542301654815673828125]
      mask Display: e = 0.06;c1 = [120 150 230]/255;c2 = ([120 150 230]+0)/383;c3 = ([120 150 230]+128)/383;patch([0 1 1 0],[0 0 1 1],c1);patch([0 1 1 1-e 1-e 0+e],[0 0 1 1-e 0+e 0+e],c2);patch([0 0 1 1-e 0+e 0+e],[0 1 1 1-e 1-e 0+e],c3);plot([0 1 1 0 0],[0 0 1 1 0]);disp('b');
  netsum : Sum  Inputs=2  InputSameDT=on  SaturateOnIntegerOverflow=on  OutDataTypeStr=Inherit: Same as first input
      mask Display: e = 0.06;c1 = [120 150 230]/255;c2 = ([120 150 230]+0)/383;c3 = ([120 150 230]+128)/383;patch([0 1 1 0],[0 0 1 1],c1);patch([0 1 1 1-e 1-e 0+e],[0 0 1 1-e 0+e 0+e],c2);patch([0 0 1 1-e 0+e 0+e],[0 1 1 1-e 1-e 0+e],c3);plot([0 1 1 0 0],[0 0 1 1 0]);disp('+');
  tansig : neural/Transfer Functions/tansig
  "a{1}" : Outport  InitialOutput=[0;0;0;0;0;0;0;0]
      mask Display: e = 0.06;c1 = [120 230 180]/255;c2 = ([120 230 180]+0)/(256+128);c3 = ([120 230 180]+128)/(256+128);patch([0 1 1 0],[0 0 1 1],c1);patch([0 1 1 1-e 1-e 0+e],[0 0 1 1-e 0+e 0+e],c2);patch([0 0 1 1-e 0+e 0+e],[0 1 1 1-e 1-e 0+e],c3);plot([0 1 1 0 0],[0 0 1 1 0]);
  wires:
  "p{1}"/1 -> Delays 1/1("p{1}")
  Delays 1/1("pd{1,1}") -> "IW{1,1}"/1("pd{1,1}")
  "IW{1,1}"/1("iz{1,1}") -> netsum/1
  "b{1}"/1 -> netsum/2
  netsum/1 -> tansig/1
  tansig/1 -> "a{1}"/1

== system three_robot_cluster_all_primitives/RGB to HSV to vel - all robots/Hue Neural Network/Layer 2 ==
  "a{1} " : Inport  PortDimensions=8
      mask Display: e = 0.06;c1 = [120 230 180]/255;c2 = ([120 230 180]+0)/(256+128);c3 = ([120 230 180]+128)/(256+128);patch([0 1 1 0],[0 0 1 1],c1);patch([0 1 1 1-e 1-e 0+e],[0 0 1 1-e 0+e 0+e],c2);patch([0 0 1 1-e 0+e 0+e],[0 1 1 1-e 1-e 0+e],c3);plot([0 1 1 0 0],[0 0 1 1 0]);
  Delays 1 : Subsystem
      mask Display: e = 0.06;c1 = [120 150 230]/255;c2 = ([120 150 230]+0)/383;c3 = ([120 150 230]+128)/383;patch([0 1 1 0],[0 0 1 1],c1);patch([0 1 1 1-e 1-e 0+e],[0 0 1 1-e 0+e 0+e],c2);patch([0 0 1 1-e 0+e 0+e],[0 1 1 1-e 1-e 0+e],c3);plot([0 1 1 0 0],[0 0 1 1 0]);disp('0');
  "LW{2,1}" : Subsystem
      mask Display: e = 0.06;c1 = [120 150 230]/255;c2 = ([120 150 230]+0)/383;c3 = ([120 150 230]+128)/383;patch([0 1 1 0],[0 0 1 1],c1);patch([0 1 1 1-e 1-e 0+e],[0 0 1 1-e 0+e 0+e],c2);patch([0 0 1 1-e 0+e 0+e],[0 1 1 1-e 1-e 0+e],c3);plot([0 1 1 0 0],[0 0 1 1 0]);disp('W');
  "b{2}" : Constant  Value=[0.675142702354909030049157081521116197109222412109375;44.9079377850743384215093101374804973602294921875;-7.0969210448822508396915509365499019622802734375;8.869391656285753100519286817871034145355224609375;-5.80408608179083795874930729041807353496551513671875;-6.54625194561882306487632376956753432750701904296875;4.23480857007052957641235479968599975109100341796875]
      mask Display: e = 0.06;c1 = [120 150 230]/255;c2 = ([120 150 230]+0)/383;c3 = ([120 150 230]+128)/383;patch([0 1 1 0],[0 0 1 1],c1);patch([0 1 1 1-e 1-e 0+e],[0 0 1 1-e 0+e 0+e],c2);patch([0 0 1 1-e 0+e 0+e],[0 1 1 1-e 1-e 0+e],c3);plot([0 1 1 0 0],[0 0 1 1 0]);disp('b');
  netsum : Sum  Inputs=2  InputSameDT=on  SaturateOnIntegerOverflow=on  OutDataTypeStr=Inherit: Same as first input
      mask Display: e = 0.06;c1 = [120 150 230]/255;c2 = ([120 150 230]+0)/383;c3 = ([120 150 230]+128)/383;patch([0 1 1 0],[0 0 1 1],c1);patch([0 1 1 1-e 1-e 0+e],[0 0 1 1-e 0+e 0+e],c2);patch([0 0 1 1-e 0+e 0+e],[0 1 1 1-e 1-e 0+e],c3);plot([0 1 1 0 0],[0 0 1 1 0]);disp('+');
  tansig : neural/Transfer Functions/tansig
  "a{2}" : Outport  InitialOutput=[0;0;0;0;0;0;0]
      mask Display: e = 0.06;c1 = [120 230 180]/255;c2 = ([120 230 180]+0)/(256+128);c3 = ([120 230 180]+128)/(256+128);patch([0 1 1 0],[0 0 1 1],c1);patch([0 1 1 1-e 1-e 0+e],[0 0 1 1-e 0+e 0+e],c2);patch([0 0 1 1-e 0+e 0+e],[0 1 1 1-e 1-e 0+e],c3);plot([0 1 1 0 0],[0 0 1 1 0]);
  wires:
  "a{1} "/1 -> Delays 1/1("p{2}")
  Delays 1/1("pd{2,1}") -> "LW{2,1}"/1("ad{2,1}")
  "LW{2,1}"/1("lz{2,1}") -> netsum/1
  "b{2}"/1 -> netsum/2
  netsum/1 -> tansig/1
  tansig/1 -> "a{2}"/1

== system three_robot_cluster_all_primitives/RGB to HSV to vel - all robots/Hue Neural Network/Layer 3 ==
  "a{2} " : Inport  PortDimensions=7
      mask Display: e = 0.06;c1 = [120 230 180]/255;c2 = ([120 230 180]+0)/(256+128);c3 = ([120 230 180]+128)/(256+128);patch([0 1 1 0],[0 0 1 1],c1);patch([0 1 1 1-e 1-e 0+e],[0 0 1 1-e 0+e 0+e],c2);patch([0 0 1 1-e 0+e 0+e],[0 1 1 1-e 1-e 0+e],c3);plot([0 1 1 0 0],[0 0 1 1 0]);
  Delays 1 : Subsystem
      mask Display: e = 0.06;c1 = [120 150 230]/255;c2 = ([120 150 230]+0)/383;c3 = ([120 150 230]+128)/383;patch([0 1 1 0],[0 0 1 1],c1);patch([0 1 1 1-e 1-e 0+e],[0 0 1 1-e 0+e 0+e],c2);patch([0 0 1 1-e 0+e 0+e],[0 1 1 1-e 1-e 0+e],c3);plot([0 1 1 0 0],[0 0 1 1 0]);disp('0');
  "LW{3,2}" : Subsystem
      mask Display: e = 0.06;c1 = [120 150 230]/255;c2 = ([120 150 230]+0)/383;c3 = ([120 150 230]+128)/383;patch([0 1 1 0],[0 0 1 1],c1);patch([0 1 1 1-e 1-e 0+e],[0 0 1 1-e 0+e 0+e],c2);patch([0 0 1 1-e 0+e 0+e],[0 1 1 1-e 1-e 0+e],c3);plot([0 1 1 0 0],[0 0 1 1 0]);disp('W');
  "b{3}" : Constant  Value=[-0.278399072270929526240479390253312885761260986328125;0.1991484574873611801404393872871878556907176971435546875]
      mask Display: e = 0.06;c1 = [120 150 230]/255;c2 = ([120 150 230]+0)/383;c3 = ([120 150 230]+128)/383;patch([0 1 1 0],[0 0 1 1],c1);patch([0 1 1 1-e 1-e 0+e],[0 0 1 1-e 0+e 0+e],c2);patch([0 0 1 1-e 0+e 0+e],[0 1 1 1-e 1-e 0+e],c3);plot([0 1 1 0 0],[0 0 1 1 0]);disp('b');
  netsum : Sum  Inputs=2  InputSameDT=on  SaturateOnIntegerOverflow=on  OutDataTypeStr=Inherit: Same as first input
      mask Display: e = 0.06;c1 = [120 150 230]/255;c2 = ([120 150 230]+0)/383;c3 = ([120 150 230]+128)/383;patch([0 1 1 0],[0 0 1 1],c1);patch([0 1 1 1-e 1-e 0+e],[0 0 1 1-e 0+e 0+e],c2);patch([0 0 1 1-e 0+e 0+e],[0 1 1 1-e 1-e 0+e],c3);plot([0 1 1 0 0],[0 0 1 1 0]);disp('+');
  purelin : neural/Transfer Functions/purelin
  "a{3}" : Outport  InitialOutput=[0;0]
      mask Display: e = 0.06;c1 = [120 230 180]/255;c2 = ([120 230 180]+0)/(256+128);c3 = ([120 230 180]+128)/(256+128);patch([0 1 1 0],[0 0 1 1],c1);patch([0 1 1 1-e 1-e 0+e],[0 0 1 1-e 0+e 0+e],c2);patch([0 0 1 1-e 0+e 0+e],[0 1 1 1-e 1-e 0+e],c3);plot([0 1 1 0 0],[0 0 1 1 0]);
  wires:
  "a{2} "/1 -> Delays 1/1("p{3}")
  Delays 1/1("pd{3,2}") -> "LW{3,2}"/1("ad{3,2}")
  "LW{3,2}"/1("lz{3,2}") -> netsum/1
  "b{3}"/1 -> netsum/2
  netsum/1 -> purelin/1
  purelin/1 -> "a{3}"/1

== system three_robot_cluster_all_primitives/RGB to HSV to vel - all robots/Hue Neural Network/Process Input 1 ==
  x : Inport  PortDimensions=4
      mask Display: e = 0.06;c1 = [120 230 180]/255;c2 = ([120 230 180]+0)/(256+128);c3 = ([120 230 180]+128)/(256+128);patch([0 1 1 0],[0 0 1 1],c1);patch([0 1 1 1-e 1-e 0+e],[0 0 1 1-e 0+e 0+e],c2);patch([0 0 1 1-e 0+e 0+e],[0 1 1 1-e 1-e 0+e],c3);plot([0 1 1 0 0],[0 0 1 1 0]);
  mapminmax : neural/Processing Functions/mapminmax  xmin=[-0.958461538461538475885959087464;-0.887692307692307669420017646189;-0.870769230769230739852559963765;-0.962857142857142855874030829]  xmax=[1;1;1;0.951999999999999957367435854394]  ymin=-1  ymax=1
  p : Outport  PortDimensions=4
      mask Display: e = 0.06;c1 = [120 230 180]/255;c2 = ([120 230 180]+0)/(256+128);c3 = ([120 230 180]+128)/(256+128);patch([0 1 1 0],[0 0 1 1],c1);patch([0 1 1 1-e 1-e 0+e],[0 0 1 1-e 0+e 0+e],c2);patch([0 0 1 1-e 0+e 0+e],[0 1 1 1-e 1-e 0+e],c3);plot([0 1 1 0 0],[0 0 1 1 0]);
  wires:
  x/1 -> mapminmax/1
  mapminmax/1 -> p/1

== system three_robot_cluster_all_primitives/RGB to HSV to vel - all robots/Hue Neural Network/Process Output 1 ==
  a : Inport  PortDimensions=2
      mask Display: e = 0.06;c1 = [120 230 180]/255;c2 = ([120 230 180]+0)/(256+128);c3 = ([120 230 180]+128)/(256+128);patch([0 1 1 0],[0 0 1 1],c1);patch([0 1 1 1-e 1-e 0+e],[0 0 1 1-e 0+e 0+e],c2);patch([0 0 1 1-e 0+e 0+e],[0 1 1 1-e 1-e 0+e],c3);plot([0 1 1 0 0],[0 0 1 1 0]);
  mapminmax_reverse : neural/Processing Functions/mapminmax_reverse  xmin=[-2.98294435394112689152734674281;-2.98294435394112689152734674281]  xmax=[0.982944353941127113571951667836;0.982944353941127113571951667836]  ymin=-1  ymax=1
  y : Outport  PortDimensions=2
      mask Display: e = 0.06;c1 = [120 230 180]/255;c2 = ([120 230 180]+0)/(256+128);c3 = ([120 230 180]+128)/(256+128);patch([0 1 1 0],[0 0 1 1],c1);patch([0 1 1 1-e 1-e 0+e],[0 0 1 1-e 0+e 0+e],c2);patch([0 0 1 1-e 0+e 0+e],[0 1 1 1-e 1-e 0+e],c3);plot([0 1 1 0 0],[0 0 1 1 0]);
  wires:
  a/1 -> mapminmax_reverse/1
  mapminmax_reverse/1 -> y/1

== system three_robot_cluster_all_primitives/RGB to HSV to vel - all robots/Sat Neural Network/Layer 1 ==
  "p{1}" : Inport  PortDimensions=4
      mask Display: e = 0.06;c1 = [120 230 180]/255;c2 = ([120 230 180]+0)/(256+128);c3 = ([120 230 180]+128)/(256+128);patch([0 1 1 0],[0 0 1 1],c1);patch([0 1 1 1-e 1-e 0+e],[0 0 1 1-e 0+e 0+e],c2);patch([0 0 1 1-e 0+e 0+e],[0 1 1 1-e 1-e 0+e],c3);plot([0 1 1 0 0],[0 0 1 1 0]);
  Delays 1 : Subsystem
      mask Display: e = 0.06;c1 = [120 150 230]/255;c2 = ([120 150 230]+0)/383;c3 = ([120 150 230]+128)/383;patch([0 1 1 0],[0 0 1 1],c1);patch([0 1 1 1-e 1-e 0+e],[0 0 1 1-e 0+e 0+e],c2);patch([0 0 1 1-e 0+e 0+e],[0 1 1 1-e 1-e 0+e],c3);plot([0 1 1 0 0],[0 0 1 1 0]);disp('0');
  "IW{1,1}" : Subsystem
      mask Display: e = 0.06;c1 = [120 150 230]/255;c2 = ([120 150 230]+0)/383;c3 = ([120 150 230]+128)/383;patch([0 1 1 0],[0 0 1 1],c1);patch([0 1 1 1-e 1-e 0+e],[0 0 1 1-e 0+e 0+e],c2);patch([0 0 1 1-e 0+e 0+e],[0 1 1 1-e 1-e 0+e],c3);plot([0 1 1 0 0],[0 0 1 1 0]);disp('W');
  "b{1}" : Constant  Value=[-2.3130522605783454537231591530144214630126953125;1.962089340663722314417327652336098253726959228515625;-1.058739181082669400524309821776114404201507568359375;-1.607608651002901734017314083757810294628143310546875;-0.7552232219962373704902347526513040065765380859375;0.28004017589954488531844845056184567511081695556640625;-0.98429304431835207278567168032168410718441009521484375;0.06645020645414635718228879568414413370192050933837890625;0.03482724950302251709643996946397237479686737060546875;1.1544893333171344362853005804936401546001434326171875;-0.86746918121114913180491612365585751831531524658203125;-1.328492664661899969047453851089812815189361572265625;-1.5286646531854219954738027809071354568004608154296875;2.027160614501038349288819517823867499828338623046875;3.18830142288625584257033551693893969058990478515625;2.82128869742971488676630542613565921783447265625]
      mask Display: e = 0.06;c1 = [120 150 230]/255;c2 = ([120 150 230]+0)/383;c3 = ([120 150 230]+128)/383;patch([0 1 1 0],[0 0 1 1],c1);patch([0 1 1 1-e 1-e 0+e],[0 0 1 1-e 0+e 0+e],c2);patch([0 0 1 1-e 0+e 0+e],[0 1 1 1-e 1-e 0+e],c3);plot([0 1 1 0 0],[0 0 1 1 0]);disp('b');
  netsum : Sum  Inputs=2  InputSameDT=on  SaturateOnIntegerOverflow=on  OutDataTypeStr=Inherit: Same as first input
      mask Display: e = 0.06;c1 = [120 150 230]/255;c2 = ([120 150 230]+0)/383;c3 = ([120 150 230]+128)/383;patch([0 1 1 0],[0 0 1 1],c1);patch([0 1 1 1-e 1-e 0+e],[0 0 1 1-e 0+e 0+e],c2);patch([0 0 1 1-e 0+e 0+e],[0 1 1 1-e 1-e 0+e],c3);plot([0 1 1 0 0],[0 0 1 1 0]);disp('+');
  tansig : neural/Transfer Functions/tansig
  "a{1}" : Outport  InitialOutput=[0;0;0;0;0;0;0;0;0;0;0;0;0;0;0;0]
      mask Display: e = 0.06;c1 = [120 230 180]/255;c2 = ([120 230 180]+0)/(256+128);c3 = ([120 230 180]+128)/(256+128);patch([0 1 1 0],[0 0 1 1],c1);patch([0 1 1 1-e 1-e 0+e],[0 0 1 1-e 0+e 0+e],c2);patch([0 0 1 1-e 0+e 0+e],[0 1 1 1-e 1-e 0+e],c3);plot([0 1 1 0 0],[0 0 1 1 0]);
  wires:
  "p{1}"/1 -> Delays 1/1("p{1}")
  Delays 1/1("pd{1,1}") -> "IW{1,1}"/1("pd{1,1}")
  "IW{1,1}"/1("iz{1,1}") -> netsum/1
  "b{1}"/1 -> netsum/2
  netsum/1 -> tansig/1
  tansig/1 -> "a{1}"/1

== system three_robot_cluster_all_primitives/RGB to HSV to vel - all robots/Sat Neural Network/Layer 2 ==
  "a{1} " : Inport  PortDimensions=16
      mask Display: e = 0.06;c1 = [120 230 180]/255;c2 = ([120 230 180]+0)/(256+128);c3 = ([120 230 180]+128)/(256+128);patch([0 1 1 0],[0 0 1 1],c1);patch([0 1 1 1-e 1-e 0+e],[0 0 1 1-e 0+e 0+e],c2);patch([0 0 1 1-e 0+e 0+e],[0 1 1 1-e 1-e 0+e],c3);plot([0 1 1 0 0],[0 0 1 1 0]);
  Delays 1 : Subsystem
      mask Display: e = 0.06;c1 = [120 150 230]/255;c2 = ([120 150 230]+0)/383;c3 = ([120 150 230]+128)/383;patch([0 1 1 0],[0 0 1 1],c1);patch([0 1 1 1-e 1-e 0+e],[0 0 1 1-e 0+e 0+e],c2);patch([0 0 1 1-e 0+e 0+e],[0 1 1 1-e 1-e 0+e],c3);plot([0 1 1 0 0],[0 0 1 1 0]);disp('0');
  "LW{2,1}" : Subsystem
      mask Display: e = 0.06;c1 = [120 150 230]/255;c2 = ([120 150 230]+0)/383;c3 = ([120 150 230]+128)/383;patch([0 1 1 0],[0 0 1 1],c1);patch([0 1 1 1-e 1-e 0+e],[0 0 1 1-e 0+e 0+e],c2);patch([0 0 1 1-e 0+e 0+e],[0 1 1 1-e 1-e 0+e],c3);plot([0 1 1 0 0],[0 0 1 1 0]);disp('W');
  "b{2}" : Constant  Value=[-1.5093043215334336348831811847048811614513397216796875;-1.3138601808265748527304594972520135343074798583984375;1.2962058200073622860060140737914480268955230712890625;0.28261103667278231199588844901882112026214599609375;-0.224969234917357263636716879773302935063838958740234375;-0.052062198356933563070381154602728202007710933685302734375;-0.504126529110695553725918216514401137828826904296875;-1.0219308132137261413419082600739784538745880126953125;-1.1221023832475374160111414312268607318401336669921875;-1.153963098850862678546036477200686931610107421875;1.546868468939315288679381410474888980388641357421875]
      mask Display: e = 0.06;c1 = [120 150 230]/255;c2 = ([120 150 230]+0)/383;c3 = ([120 150 230]+128)/383;patch([0 1 1 0],[0 0 1 1],c1);patch([0 1 1 1-e 1-e 0+e],[0 0 1 1-e 0+e 0+e],c2);patch([0 0 1 1-e 0+e 0+e],[0 1 1 1-e 1-e 0+e],c3);plot([0 1 1 0 0],[0 0 1 1 0]);disp('b');
  netsum : Sum  Inputs=2  InputSameDT=on  SaturateOnIntegerOverflow=on  OutDataTypeStr=Inherit: Same as first input
      mask Display: e = 0.06;c1 = [120 150 230]/255;c2 = ([120 150 230]+0)/383;c3 = ([120 150 230]+128)/383;patch([0 1 1 0],[0 0 1 1],c1);patch([0 1 1 1-e 1-e 0+e],[0 0 1 1-e 0+e 0+e],c2);patch([0 0 1 1-e 0+e 0+e],[0 1 1 1-e 1-e 0+e],c3);plot([0 1 1 0 0],[0 0 1 1 0]);disp('+');
  tansig : neural/Transfer Functions/tansig
  "a{2}" : Outport  InitialOutput=[0;0;0;0;0;0;0;0;0;0;0]
      mask Display: e = 0.06;c1 = [120 230 180]/255;c2 = ([120 230 180]+0)/(256+128);c3 = ([120 230 180]+128)/(256+128);patch([0 1 1 0],[0 0 1 1],c1);patch([0 1 1 1-e 1-e 0+e],[0 0 1 1-e 0+e 0+e],c2);patch([0 0 1 1-e 0+e 0+e],[0 1 1 1-e 1-e 0+e],c3);plot([0 1 1 0 0],[0 0 1 1 0]);
  wires:
  "a{1} "/1 -> Delays 1/1("p{2}")
  Delays 1/1("pd{2,1}") -> "LW{2,1}"/1("ad{2,1}")
  "LW{2,1}"/1("lz{2,1}") -> netsum/1
  "b{2}"/1 -> netsum/2
  netsum/1 -> tansig/1
  tansig/1 -> "a{2}"/1

== system three_robot_cluster_all_primitives/RGB to HSV to vel - all robots/Sat Neural Network/Layer 3 ==
  "a{2} " : Inport  PortDimensions=11
      mask Display: e = 0.06;c1 = [120 230 180]/255;c2 = ([120 230 180]+0)/(256+128);c3 = ([120 230 180]+128)/(256+128);patch([0 1 1 0],[0 0 1 1],c1);patch([0 1 1 1-e 1-e 0+e],[0 0 1 1-e 0+e 0+e],c2);patch([0 0 1 1-e 0+e 0+e],[0 1 1 1-e 1-e 0+e],c3);plot([0 1 1 0 0],[0 0 1 1 0]);
  Delays 1 : Subsystem
      mask Display: e = 0.06;c1 = [120 150 230]/255;c2 = ([120 150 230]+0)/383;c3 = ([120 150 230]+128)/383;patch([0 1 1 0],[0 0 1 1],c1);patch([0 1 1 1-e 1-e 0+e],[0 0 1 1-e 0+e 0+e],c2);patch([0 0 1 1-e 0+e 0+e],[0 1 1 1-e 1-e 0+e],c3);plot([0 1 1 0 0],[0 0 1 1 0]);disp('0');
  "LW{3,2}" : Subsystem
      mask Display: e = 0.06;c1 = [120 150 230]/255;c2 = ([120 150 230]+0)/383;c3 = ([120 150 230]+128)/383;patch([0 1 1 0],[0 0 1 1],c1);patch([0 1 1 1-e 1-e 0+e],[0 0 1 1-e 0+e 0+e],c2);patch([0 0 1 1-e 0+e 0+e],[0 1 1 1-e 1-e 0+e],c3);plot([0 1 1 0 0],[0 0 1 1 0]);disp('W');
  "b{3}" : Constant  Value=0.85891032553784774083993625026778317987918853759765625
      mask Display: e = 0.06;c1 = [120 150 230]/255;c2 = ([120 150 230]+0)/383;c3 = ([120 150 230]+128)/383;patch([0 1 1 0],[0 0 1 1],c1);patch([0 1 1 1-e 1-e 0+e],[0 0 1 1-e 0+e 0+e],c2);patch([0 0 1 1-e 0+e 0+e],[0 1 1 1-e 1-e 0+e],c3);plot([0 1 1 0 0],[0 0 1 1 0]);disp('b');
  netsum : Sum  Inputs=2  InputSameDT=on  SaturateOnIntegerOverflow=on  OutDataTypeStr=Inherit: Same as first input
      mask Display: e = 0.06;c1 = [120 150 230]/255;c2 = ([120 150 230]+0)/383;c3 = ([120 150 230]+128)/383;patch([0 1 1 0],[0 0 1 1],c1);patch([0 1 1 1-e 1-e 0+e],[0 0 1 1-e 0+e 0+e],c2);patch([0 0 1 1-e 0+e 0+e],[0 1 1 1-e 1-e 0+e],c3);plot([0 1 1 0 0],[0 0 1 1 0]);disp('+');
  purelin : neural/Transfer Functions/purelin
  "a{3}" : Outport  InitialOutput=0
      mask Display: e = 0.06;c1 = [120 230 180]/255;c2 = ([120 230 180]+0)/(256+128);c3 = ([120 230 180]+128)/(256+128);patch([0 1 1 0],[0 0 1 1],c1);patch([0 1 1 1-e 1-e 0+e],[0 0 1 1-e 0+e 0+e],c2);patch([0 0 1 1-e 0+e 0+e],[0 1 1 1-e 1-e 0+e],c3);plot([0 1 1 0 0],[0 0 1 1 0]);
  wires:
  "a{2} "/1 -> Delays 1/1("p{3}")
  Delays 1/1("pd{3,2}") -> "LW{3,2}"/1("ad{3,2}")
  "LW{3,2}"/1("lz{3,2}") -> netsum/1
  "b{3}"/1 -> netsum/2
  netsum/1 -> purelin/1
  purelin/1 -> "a{3}"/1

== system three_robot_cluster_all_primitives/RGB to HSV to vel - all robots/Sat Neural Network/Process Input 1 ==
  x : Inport  PortDimensions=4
      mask Display: e = 0.06;c1 = [120 230 180]/255;c2 = ([120 230 180]+0)/(256+128);c3 = ([120 230 180]+128)/(256+128);patch([0 1 1 0],[0 0 1 1],c1);patch([0 1 1 1-e 1-e 0+e],[0 0 1 1-e 0+e 0+e],c2);patch([0 0 1 1-e 0+e 0+e],[0 1 1 1-e 1-e 0+e],c3);plot([0 1 1 0 0],[0 0 1 1 0]);
  mapminmax : neural/Processing Functions/mapminmax  xmin=[-0.963880974842093563026423908013;-0.895075127280099080984143711248;-0.874403186471323534689759071625;-0.998018709638442746978626018972]  xmax=[1;1;1;0.96191445593493396515327731322]  ymin=-1  ymax=1
  p : Outport  PortDimensions=4
      mask Display: e = 0.06;c1 = [120 230 180]/255;c2 = ([120 230 180]+0)/(256+128);c3 = ([120 230 180]+128)/(256+128);patch([0 1 1 0],[0 0 1 1],c1);patch([0 1 1 1-e 1-e 0+e],[0 0 1 1-e 0+e 0+e],c2);patch([0 0 1 1-e 0+e 0+e],[0 1 1 1-e 1-e 0+e],c3);plot([0 1 1 0 0],[0 0 1 1 0]);
  wires:
  x/1 -> mapminmax/1
  mapminmax/1 -> p/1
